simulink model "lab3_model_3"  (R2015a)
settings: Solver=ode4  SolverMode=SingleTasking  StartTime=0.0  StopTime=10.0  FixedStep=1e-2  RelTol=1e-3
values from neighbouring files (symbols this model uses):
  K0 = 1000    [script3.m]
  m = marr(i)    [script3.m]
  n = 24    [script3.m]
  r = 10    [script3.m]
settings Model: Creator=bb  LastModifiedBy=bb
settings DataIOCC: LimitDataPoints=off

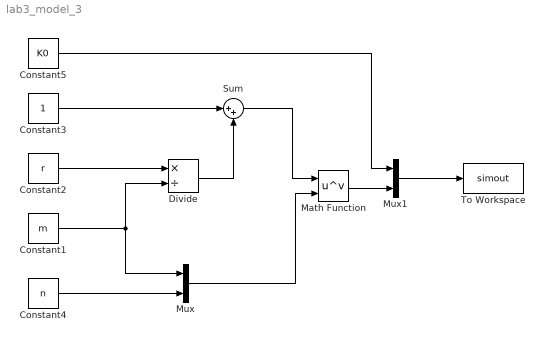
== system lab3_model_3 ==
  Constant1 : Constant  Value=m
  Constant2 : Constant  Value=r
  Constant3 : Constant
  Constant4 : Constant  Value=n
  Constant5 : Constant  Value=K0
  Divide : Product  Inputs=*/
  Math Function : Math  Operator=pow  SaturateOnIntegerOverflow=on
  Mux : Mux  Inputs=2
  Mux1 : Mux  Inputs=2
  Sum : Sum  Inputs=|++
  To Workspace : ToWorkspace  VariableName=simout  SampleTime=-1
  wires:
  Constant1/1 -> Mux/1, Divide/2
  Divide/1 -> Sum/2
  Constant3/1 -> Sum/1
  Constant2/1 -> Divide/1
  Math Function/1 -> Mux1/2
  Sum/1 -> Math Function/1
  Constant4/1 -> Mux/2
  Mux/1 -> Math Function/2
  Mux1/1 -> To Workspace/1
  Constant5/1 -> Mux1/1
